simulink model "exp4_1_sim"  (R2023b)
settings: Solver=VariableStepAuto  StartTime=0.0  StopTime=10.0  RelTol=1e-3
settings Model: Creator=27198  LastModifiedBy=27198

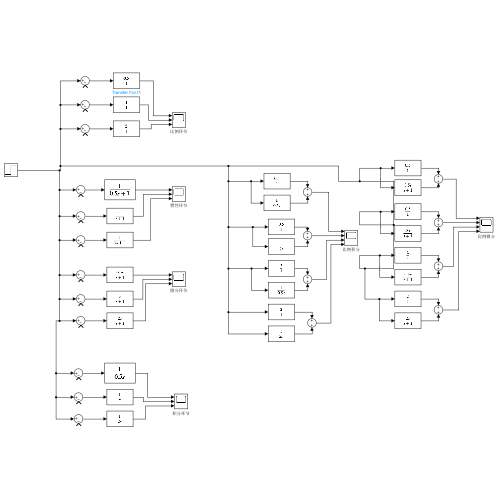
[thumbnail: Simulink's stored preview of the top-level diagram]
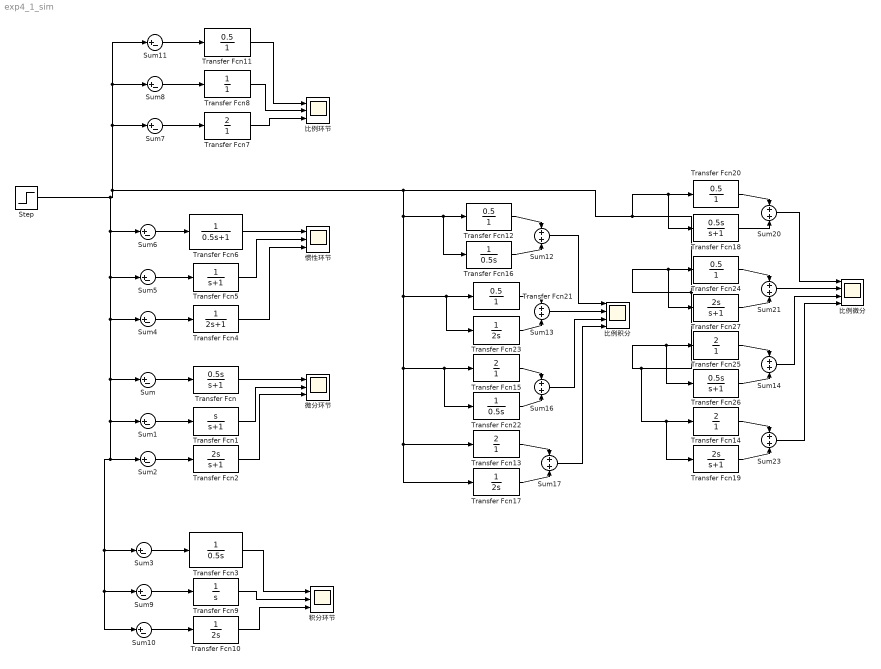
== system exp4_1_sim ==
  Step : Step  SampleTime=0
  Sum{,1..11} (12 alike) : Sum  Inputs=|+-
  Sum{12..14,16..17,20..21,23} (8 alike) : Sum
  Transfer Fcn : TransferFcn  Numerator=[0.5 0]  Denominator=[1 1]
  Transfer Fcn1 : TransferFcn  Numerator=[1 0]  Denominator=[1 1]
  Transfer Fcn10 : TransferFcn  Denominator=[2 0]
  Transfer Fcn{11..12,20..21,24} (5 alike) : TransferFcn  Numerator=[0.5]  Denominator=[1]
  Transfer Fcn{7,13..15,25} (5 alike) : TransferFcn  Numerator=[2]  Denominator=[1]
  Transfer Fcn16 : TransferFcn  Denominator=[0.5 0]
  Transfer Fcn17 : TransferFcn  Denominator=[2 0]
  Transfer Fcn18 : TransferFcn  Numerator=[0.5 0]  Denominator=[1 1]
  Transfer Fcn19 : TransferFcn  Numerator=[2 0]  Denominator=[1 1]
  Transfer Fcn2 : TransferFcn  Numerator=[2 0]  Denominator=[1 1]
  Transfer Fcn22 : TransferFcn  Denominator=[0.5 0]
  Transfer Fcn23 : TransferFcn  Denominator=[2 0]
  Transfer Fcn26 : TransferFcn  Numerator=[0.5 0]  Denominator=[1 1]
  Transfer Fcn27 : TransferFcn  Numerator=[2 0]  Denominator=[1 1]
  Transfer Fcn3 : TransferFcn  Denominator=[0.5 0]
  Transfer Fcn4 : TransferFcn  Denominator=[2 1]
  Transfer Fcn5 : TransferFcn  Denominator=[1 1]
  Transfer Fcn6 : TransferFcn  Denominator=[0.5 1]
  Transfer Fcn8 : TransferFcn  Denominator=[1]
  Transfer Fcn9 : TransferFcn  Denominator=[1 0]
  微分环节 : Scope  NumInputPorts=3
  惯性环节 : Scope  NumInputPorts=3
  比例微分 : Scope  NumInputPorts=4
  比例环节 : Scope  NumInputPorts=3
  比例积分 : Scope  NumInputPorts=4
  积分环节 : Scope  NumInputPorts=3
  wires:
  Transfer Fcn18/1 -> Sum20/2
  Transfer Fcn6/1 -> 惯性环节/1
  Sum17/1 -> 比例积分/4
  Sum2/1 -> Transfer Fcn2/1
  Transfer Fcn11/1 -> 比例环节/1
  Transfer Fcn/1 -> 微分环节/1
  Transfer Fcn5/1 -> 惯性环节/2
  Transfer Fcn23/1 -> Sum13/2
  Sum3/1 -> Transfer Fcn3/1
  Sum4/1 -> Transfer Fcn4/1
  Transfer Fcn25/1 -> Sum14/1
  Transfer Fcn2/1 -> 微分环节/3
  Sum16/1 -> 比例积分/3
  Transfer Fcn21/1 -> Sum13/1
  Sum12/1 -> 比例积分/1
  Transfer Fcn3/1 -> 积分环节/1
  Sum5/1 -> Transfer Fcn5/1
  Step/1 -> Sum11/1, Sum8/1, Sum7/1, Transfer Fcn19/1, Transfer Fcn14/1, Transfer Fcn26/1, Transfer Fcn25/1, Transfer Fcn27/1, Transfer Fcn24/1, Transfer Fcn18/1, Transfer Fcn20/1, Transfer Fcn13/1, Transfer Fcn17/1, Transfer Fcn22/1, Transfer Fcn15/1, Transfer Fcn23/1, Transfer Fcn21/1, Transfer Fcn16/1, Transfer Fcn12/1, Sum10/1, Sum9/1, Sum3/1, Sum2/1, Sum1/1, Sum/1, Sum4/1, Sum5/1, Sum6/1
  Transfer Fcn4/1 -> 惯性环节/3
  Sum13/1 -> 比例积分/2
  Transfer Fcn16/1 -> Sum12/2
  Sum9/1 -> Transfer Fcn9/1
  Sum6/1 -> Transfer Fcn6/1
  Transfer Fcn10/1 -> 积分环节/3
  Sum8/1 -> Transfer Fcn8/1
  Sum23/1 -> 比例微分/4
  Transfer Fcn1/1 -> 微分环节/2
  Transfer Fcn13/1 -> Sum17/1
  Transfer Fcn15/1 -> Sum16/1
  Transfer Fcn8/1 -> 比例环节/2
  Sum10/1 -> Transfer Fcn10/1
  Transfer Fcn24/1 -> Sum21/1
  Sum7/1 -> Transfer Fcn7/1
  Transfer Fcn20/1 -> Sum20/1
  Sum20/1 -> 比例微分/1
  Transfer Fcn27/1 -> Sum21/2
  Transfer Fcn17/1 -> Sum17/2
  Sum1/1 -> Transfer Fcn1/1
  Transfer Fcn22/1 -> Sum16/2
  Sum/1 -> Transfer Fcn/1
  Sum21/1 -> 比例微分/2
  Transfer Fcn19/1 -> Sum23/2
  Transfer Fcn7/1 -> 比例环节/3
  Transfer Fcn12/1 -> Sum12/1
  Transfer Fcn14/1 -> Sum23/1
  Sum14/1 -> 比例微分/3
  Transfer Fcn26/1 -> Sum14/2
  Transfer Fcn9/1 -> 积分环节/2
  Sum11/1 -> Transfer Fcn11/1
